simulink model "hdl_model"  (R2024a)
settings: Solver=VariableStepAuto  StartTime=0.0  StopTime=2  RelTol=1e-3
undefined symbols (not defined in the file or in its folder): BUFFER_LEN, SAMPLING_FREQ, signal_1
libraries: hdlsllib x2, dspsrcs4 x1, dsphdlxfrm2 x1, dspsigops x1, simulink x1
settings Model: SimulationMode=accelerator  Creator=Jan Rosa  LastModifiedBy=Jan Rosa

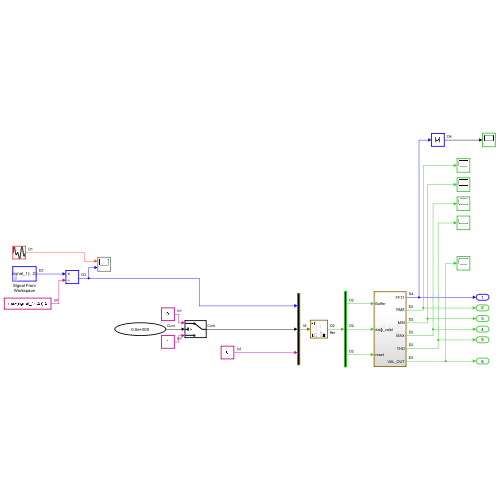
[thumbnail: Simulink's stored preview of the top-level diagram]
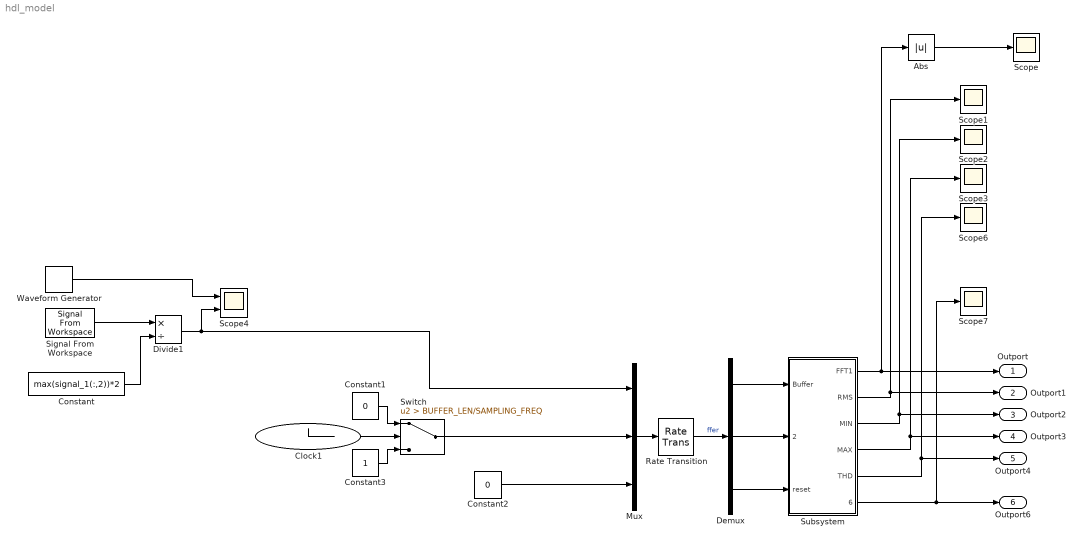
== system hdl_model ==
  Abs : Abs  SaturateOnIntegerOverflow=off
  Clock1 : Clock
  Constant : Constant  Value=max(signal_1(:,2))*2
  Constant1 : Constant  Value=0
  Constant2 : Constant  Value=0
  Constant3 : Constant
  Demux : Demux  Outputs=3
  Divide1 : Product  Inputs=*/
  Mux : Mux  Inputs=3
  Rate Transition : RateTransition  Integrity=off  Deterministic=off  OutPortSampleTime=1/SAMPLING_FREQ
  Scope{,1..3,6..7} (6 alike) : Scope
  Scope4 : Scope  NumInputPorts=2
  Signal From Workspace : dspsrcs4/Signal From Workspace  X=signal_1(:, 2)  Ts=signal_1(2, 1)  nsamps=1  OutputAfterFinalValue=Cyclic repetition  ignoreOrWarnInputAndFrameLengths=off  OutputFrames=off
  Subsystem : Subsystem
  Switch : Switch  Criteria=u2 > Threshold  Threshold=BUFFER_LEN/SAMPLING_FREQ  SaturateOnIntegerOverflow=off  InputSameDT=off
  Waveform Generator : simulink/Sources/Waveform Generator  OutMin=[]  OutMax=[]  OutDataTypeStr=double  SelectedSignal=1  Signals=0.99*sin(0.5, 50*2*pi, 0)  BlockNames=MultiportSwitch_c7ceefe4d1e8441  SampleTime=1/(SAMPLING_FREQ*2)
  Outport : Outport
  Outport1 : Outport  Port=2
  Outport2 : Outport  Port=3
  Outport3 : Outport  Port=4
  Outport4 : Outport  Port=5
  Outport6 : Outport  Port=6
  wires:
  Divide1/1 -> Mux/1, Scope4/2
  Signal From Workspace/1 -> Divide1/1
  Constant/1 -> Divide1/2
  Waveform Generator/1 -> Scope4/1
  Clock1/1 -> Switch/2
  Switch/1 -> Mux/2
  Constant3/1 -> Switch/3
  Constant2/1 -> Mux/3
  Constant1/1 -> Switch/1
  Subsystem/1(FFT1) -> Outport/1, Abs/1
  Subsystem/2(RMS) -> Outport1/1, Scope1/1
  Mux/1 -> Rate Transition/1
  Demux/1 -> Subsystem/1(Buffer)
  Demux/2 -> Subsystem/2(data_valid)
  Demux/3 -> Subsystem/3(reset)
  Rate Transition/1 -> Demux/1  "ffer"
  Subsystem/3(MIN) -> Outport2/1, Scope2/1
  Subsystem/4(MAX) -> Outport3/1, Scope3/1
  Subsystem/5(THD) -> Outport4/1, Scope6/1
  Subsystem/6(VAL_OUT) -> Outport6/1, Scope7/1
  Abs/1 -> Scope/1

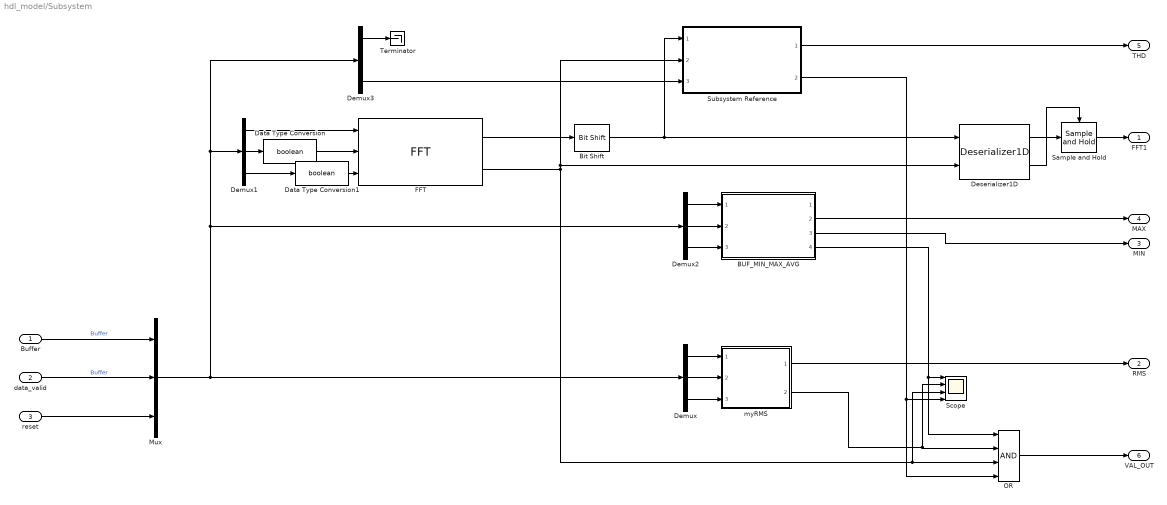
== system hdl_model/Subsystem ==
  Buffer : Inport
  data_valid : Inport  Port=2
  reset : Inport  Port=3
  BUF_MIN_MAX_AVG : Subsystem  ReferencedSubsystem=BUF_MIN_MAX_AVG
  Bit Shift : hdlsllib/Logic and Bit Operations/Bit Shift  mode=Shift Right Arithmetic  N=log2(BUFFER_LEN)
  Data Type Conversion : DataTypeConversion  OutDataTypeStr=boolean  SaturateOnIntegerOverflow=off  RndMeth=Floor
  Data Type Conversion1 : DataTypeConversion  OutDataTypeStr=boolean  SaturateOnIntegerOverflow=off  RndMeth=Floor
  Demux{,1..3} (4 alike) : Demux  Outputs=3
  Deserializer1D : hdlsllib/HDL Operations/Deserializer1D  Ratio=BUFFER_LEN  IdleCycles=0  InitialCondition=0  startIn=off  validIn=on  validOut=on  inputDataDimensions=-1  inputSampleTime=-1  inputSignalType=auto
  FFT : dsphdlxfrm2/FFT  Architecture=Streaming Radix 2^2  FFTLengthSource=Property  FFTLength=BUFFER_LEN  FFTLengthMax=1024  ComplexMultiplication=Use 4 multipliers and 2 adders  BitReversedOutput=off  BitReversedInput=off  Normalize=off  SimulateUsing=Code generation  RoundingMethod=Floor  ResetInputPort=on  StartOutputPort=off  EndOutputPort=off
  Mux : Mux  Inputs=3
  OR : Logic  Inputs=4  IconShape=distinctive  AllPortsSameDT=off  OutDataTypeStr=boolean
  Sample and Hold : dspsigops/Sample and Hold  trig=Rising edge  initCond=0  latchinput=off
  Scope : Scope  NumInputPorts=4
  Subsystem Reference : Subsystem  ReferencedSubsystem=myTHD
  Terminator : Terminator
  myRMS : Subsystem  ReferencedSubsystem=myRMS
  FFT1 : Outport
  RMS : Outport  Port=2
  MIN : Outport  Port=3
  MAX : Outport  Port=4
  THD : Outport  Port=5
  VAL_OUT : Outport  Port=6
  wires:
  OR/1 -> VAL_OUT/1
  FFT/2 -> Deserializer1D/2, Subsystem Reference/2, OR/3, Scope/3
  BUF_MIN_MAX_AVG/2 -> MAX/1
  BUF_MIN_MAX_AVG/3 -> MIN/1
  BUF_MIN_MAX_AVG/4 -> OR/1, Scope/1
  myRMS/1 -> RMS/1
  myRMS/2 -> OR/2, Scope/2
  Buffer/1 -> Mux/1  "Buffer"
  Demux/2 -> myRMS/2
  Demux/1 -> myRMS/1
  reset/1 -> Mux/3
  data_valid/1 -> Mux/2  "Buffer"
  Demux/3 -> myRMS/3
  Mux/1 -> Demux2/1, Demux3/1, Demux1/1, Demux/1
  Demux1/1 -> FFT/1
  Demux1/2 -> Data Type Conversion/1
  Demux1/3 -> Data Type Conversion1/1
  Demux2/1 -> BUF_MIN_MAX_AVG/1
  Demux2/2 -> BUF_MIN_MAX_AVG/2
  Demux2/3 -> BUF_MIN_MAX_AVG/3
  Demux3/3 -> Subsystem Reference/3
  Demux3/1 -> Terminator/1
  Subsystem Reference/1 -> THD/1
  Subsystem Reference/2 -> OR/4, Scope/4
  Data Type Conversion1/1 -> FFT/3
  Data Type Conversion/1 -> FFT/2
  Bit Shift/1 -> Subsystem Reference/1, Deserializer1D/1
  FFT/1 -> Bit Shift/1
  Deserializer1D/1 -> Sample and Hold/1
  Sample and Hold/1 -> FFT1/1
  Deserializer1D/2 -> Sample and Hold/Trigger
